simulink model "simu_sat"  (R2018b)
settings: Solver=FixedStepAuto  StartTime=0.0  StopTime=0.5  FixedStep=0.001  RelTol=1e-3
undefined symbols (not defined in the file or in its folder): sistema_velocidade
settings Model: Creator=lubuntu  LastModifiedBy=lubuntu

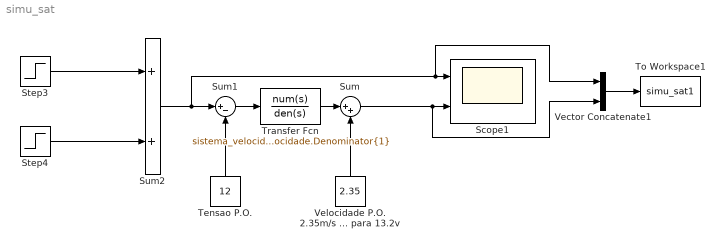
== system simu_sat ==
  Scope1 : Scope  NumInputPorts=2
  Step3 : Step  Time=0.1  Before=12  After=24  SampleTime=0
  Step4 : Step  Time=0.302  After=-12+12*0.10  SampleTime=0
  Sum : Sum  Inputs=|++
  Sum1 : Sum  Inputs=|+-
  Sum2 : Sum
  Tensao P.O. : Constant  Value=12
  To Workspace1 : ToWorkspace  VariableName=simu_sat1  SaveFormat=Timeseries  SampleTime=-1
  Transfer Fcn : TransferFcn  Numerator=sistema_velocidade.Numerator{1}  Denominator=sistema_velocidade.Denominator{1}
  Vector Concatenate1 : Concatenate
  Velocidade P.O. 2.35m/s para 12v 2.59m/s para 13.2v : Constant  Value=2.35
  wires:
  Step4/1 -> Sum2/2
  Vector Concatenate1/1 -> To Workspace1/1
  Step3/1 -> Sum2/1
  Transfer Fcn/1 -> Sum/1
  Sum/1 -> Vector Concatenate1/2, Scope1/2
  Velocidade P.O. 2.35m/s para 12v 2.59m/s para 13.2v/1 -> Sum/2
  Sum2/1 -> Sum1/1, Vector Concatenate1/1, Scope1/1
  Sum1/1 -> Transfer Fcn/1
  Tensao P.O./1 -> Sum1/2
